simulink model "modelisation_nacelle_pour_tp_moteur_2015b"  (R2015b)
settings: Solver=VariableStepAuto  StartTime=0.0  StopTime=10  RelTol=1e-3
PreLoadFcn:
  | coef_ff=0.002
  | L=0.012
  | R=11
  | Ualim=7.2
  | kw=2e-2
  | p=7
  | echelon_roulis=10
  | echelon_tangage=10
  | kp_roulis=1000
  | ki_roulis=800
  | kd_roulis=0
  | kp_tangage=1000
  | ki_tangage=800
  | kd_tangage=0
  | pwm_max=127
undefined symbols (not defined in the file): sigbuilder_block, X, Y, Z
libraries: sm_lib x164, nesl_utility x5, simulink x1
(part 1 of 4)
settings Model: Creator=pt_ptsi  LastModifiedBy=Phil
settings SolverCC: ZeroCrossAlgorithm=Adaptive
settings DataIOCC: SaveFormat=Array
settings OptimizationCC: ExpressionDepthLimit=2147483647
settings DebuggingCC: UnderspecifiedInitializationDetection=Classic  MergeDetectMultiDrivingBlocksExec=none  SolverPrmCheckMsg=warning  StateNameClashWarn=warning
settings HardwareCC: ProdBitPerPointer=32  ProdLargestAtomicFloat=None  ProdIntDivRoundTo=Undefined  ProdEndianess=Unspecified  ProdWordSize=32  ProdHWDeviceType=32-bit Generic
settings GRTTargetCC: GeneratePreprocessorConditionals=Disable all
settings ConfigComp: CovModelRefEnable=Off
settings ExplorerConfigSet: SimMechanicsOpenEditorOnUpdate=off  InternalSimMechanicsExplorerSettings="<ExplorerConfiguration><canonicalview>default</canonicalview><AnimationSetting><BasePlaybackSpeed>1.0</BasePlaybackSpeed><PlaybackSpeedFactor>1.0</PlaybackSpeedFactor></AnimationSetting><TilePanel><TileInfo><Tiles Columns=\"1\" Count=\"1\" Rows=\"1\"><Column Left=\"2\" Weight=\"1\"/><Column Left=\"662\"/><Row Top=\"2\" Weight=\"1\"/><Row Top=\"396\"/><Tile Height=\"1\" Width=\"1\" X=\"0\" Y=\"0\"/></Tiles></TileInfo><SceneInfo><SceneViewer><BGColor><R>0.60000002384185791</R><G>0.60000002384185791</G><B>0.60000002384185791</B></BGColor><Camera><DoPerspective>off</DoPerspective><Position><X>12.213943667440395</X><Y>12.912141479051609</Y><Z>-9.9128663307728146</Z></Position><Center><X>0.0036568356529240731</X><Y>0.0029282546692730449</Y><Z>-0.080202307970983711</Z></Center><Up><X>0.79405149944444098</X><Y>-0.40757170789975361</Y><Z>0.45096288001310419</Z></Up><ViewLimDist>1</ViewLimDist><YLim>0.061319680660963063</YLim><XLim>0.10368600548126482</XLim></Camera></SceneViewer></SceneInfo></TilePanel><MechEditorPanel><Cameras/><GfxPanelCameraMap/></MechEditorPanel></ExplorerConfiguration>"

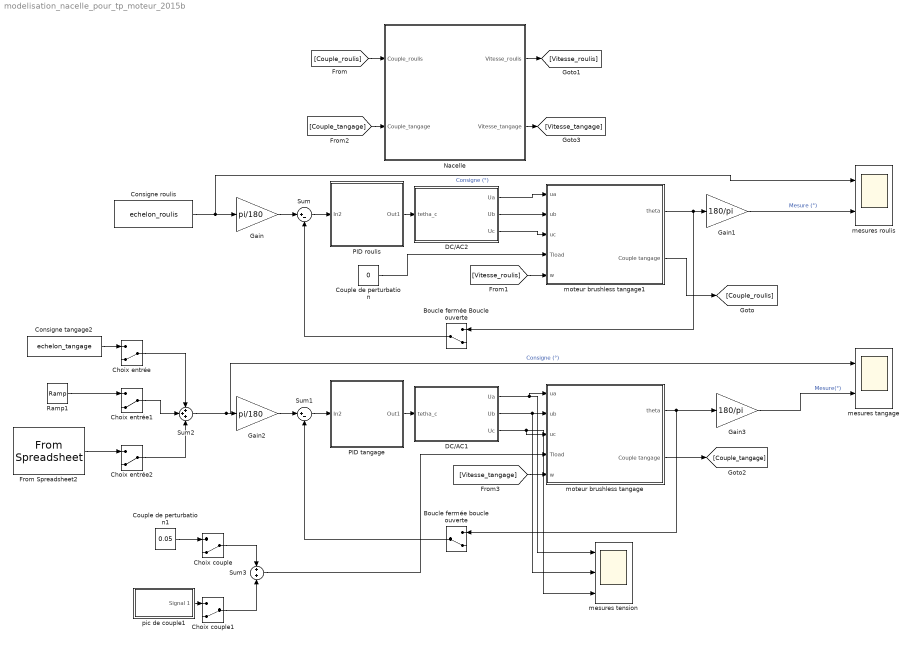
== system modelisation_nacelle_pour_tp_moteur_2015b ==
  Boucle fermée Boucle ouverte : ManualSwitch  CurrentSetting=0
  Boucle fermée boucle ouverte : ManualSwitch  CurrentSetting=0
  Choix couple : ManualSwitch  CurrentSetting=0
  Choix couple1 : ManualSwitch  CurrentSetting=0
  Choix entrée : ManualSwitch  CurrentSetting=0
  Choix entrée1 : ManualSwitch  CurrentSetting=0
  Choix entrée2 : ManualSwitch  CurrentSetting=0
  Consigne roulis : Constant  Value=echelon_roulis
  Consigne tangage2 : Constant  Value=echelon_tangage
  Couple de perturbation : Constant  Value=0
  Couple de perturbation1 : Constant  Value=0.05
  DC/AC1 : Subsystem
      mask Display: image('DC_AC.bmp')
  DC/AC2 : Subsystem
      mask Display: image('DC_AC.bmp')
  From Spreadsheet2 : FromSpreadsheet  FileName=pos.xlsx  SheetName=Feuil1
  Gain : Gain  Gain=pi/180
  Gain1 : Gain  Gain=180/pi
  Gain2 : Gain  Gain=pi/180
  Gain3 : Gain  Gain=180/pi
  Nacelle : Subsystem
      mask Display: image('image_nacelle.bmp')
  PID roulis : Subsystem
      mask Display: image('image PID.bmp')
  PID tangage : Subsystem
      mask Display: image('image PID.bmp')
  Ramp1 : simulink/Sources/Ramp  slope=100  start=0  X0=0
  Sum : Sum  Inputs=|+-
  Sum1 : Sum  Inputs=|+-
  Sum2 : Sum  Inputs=+++
  Sum3 : Sum
  mesures roulis : Scope  NumInputPorts=2
  mesures tangage : Scope  NumInputPorts=2
  mesures tension : Scope  NumInputPorts=3
  moteur brushless tangage : Subsystem
      mask Display: image('moteurBL.jpg')
  moteur brushless tangage1 : Subsystem
      mask Display: image('moteurBL.jpg')
  pic de couple1 : Subsystem  Tag=STV Subsys  LoadFcn=sigbuilder_block('load');  StartFcn=sigbuilder_block('start');  StopFcn=sigbuilder_block('stop');  ClipboardFcn=sigbuilder_block('clipboard');  mask(Sigbuilder block){}
      mask help: Simulink:masks:SigbuilderBlock_MD
      mask init:
      | if ~strcmp(get_param(bdroot(gcbh),'SimulationStatus'),'stopped') tuvar = sigbuilder_block('maskInit'); end
      settings: CopyFcn=sigbuilder_block('copy');  DeleteFcn=sigbuilder_block('delete');  ModelCloseFcn=sigbuilder_block('modelClose');  PreSaveFcn=sigbuilder_block('preSave');  PauseFcn=sigbuilder_block('pause');  ContinueFcn=sigbuilder_block('continue');  NameChangeFcn=sigbuilder_block('namechange');  OpenFcn=sigbuilder_block('open',[6 30 1428 682.5 ]);  CloseFcn=sigbuilder_block('close');
      mask Display: plot(0, 0, 100, 100,[2, 2, 32, 32, 2], [68, 8, 8, 68, 68],[32, 2], [38, 38], [32, 19, 2],[53, 60, 44], [32, 17, 17, 2],[16, 16, 31, 31]);txt = getActiveGroup(gcbh);text(2, 100, txt,'verticalAlignment', 'top');
  wires:
  DC/AC2/1(Ua) -> moteur brushless tangage1/1(ua)
  DC/AC2/2(Ub) -> moteur brushless tangage1/2(ub)
  DC/AC2/3(Uc) -> moteur brushless tangage1/3(uc)
  Couple de perturbation/1 -> moteur brushless tangage1/4(Tload)
  Gain/1 -> Sum/1
  moteur brushless tangage1/1(theta) -> Boucle fermée Boucle ouverte/1, Gain1/1
  Boucle fermée Boucle ouverte/1 -> Sum/2
  Consigne roulis/1 -> Gain/1, mesures roulis/1  "Consigne (°)"
  Gain1/1 -> mesures roulis/2  "Mesure (°)"
  Sum/1 -> PID roulis/1(In2)
  PID roulis/1(Out1) -> DC/AC2/1(tetha_c)
  Gain2/1 -> Sum1/1
  moteur brushless tangage/1(theta) -> Boucle fermée boucle ouverte/1, Gain3/1
  Boucle fermée boucle ouverte/1 -> Sum1/2
  Sum2/1 -> Gain2/1, mesures tangage/1  "Consigne (°)"
  Gain3/1 -> mesures tangage/2  "Mesure(°)"
  DC/AC1/1(Ua) -> mesures tension/1, moteur brushless tangage/1(ua)
  DC/AC1/2(Ub) -> mesures tension/2, moteur brushless tangage/2(ub)
  DC/AC1/3(Uc) -> mesures tension/3, moteur brushless tangage/3(uc)
  Sum1/1 -> PID tangage/1(In2)
  PID tangage/1(Out1) -> DC/AC1/1(tetha_c)
  moteur brushless tangage1/2(Couple tangage) -> [Couple_roulis]
  [Couple_roulis] -> Nacelle/1(Couple_roulis)
  [Vitesse_roulis] -> moteur brushless tangage1/5(w)
  Nacelle/1(Vitesse_roulis) -> [Vitesse_roulis]
  moteur brushless tangage/2(Couple tangage) -> [Couple_tangage]
  [Couple_tangage] -> Nacelle/2(Couple_tangage)
  Nacelle/2(Vitesse_tangage) -> [Vitesse_tangage]
  [Vitesse_tangage] -> moteur brushless tangage/5(w)
  Sum3/1 -> moteur brushless tangage/4(Tload)
  Consigne tangage2/1 -> Choix entrée/1
  Ramp1/1 -> Choix entrée1/1
  From Spreadsheet2/1 -> Choix entrée2/1
  Choix entrée/1 -> Sum2/1
  Choix entrée1/1 -> Sum2/2
  Choix entrée2/1 -> Sum2/3
  Couple de perturbation1/1 -> Choix couple/1
  pic de couple1/1(Signal 1) -> Choix couple1/1
  Choix couple1/1 -> Sum3/2
  Choix couple/1 -> Sum3/1

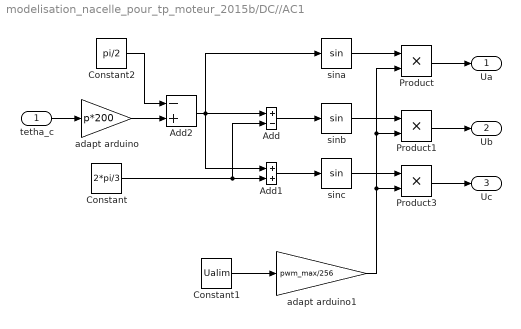
== system modelisation_nacelle_pour_tp_moteur_2015b/DC//AC1 ==
  tetha_c : Inport
  Add : Sum  Inputs=+-
  Add1 : Sum
  Add2 : Sum  Inputs=-+
  Constant : Constant  Value=2*pi/3
  Constant1 : Constant  Value=Ualim
  Constant2 : Constant  Value=pi/2
  Product : Product  RndMeth=Zero
  Product1 : Product  RndMeth=Zero
  Product3 : Product  RndMeth=Zero
  adapt arduino : Gain  Gain=p*200
  adapt arduino1 : Gain  Gain=pwm_max/256
  sina : Trigonometry
  sinb : Trigonometry
  sinc : Trigonometry
  Ua : Outport
  Ub : Outport  Port=2
  Uc : Outport  Port=3
  wires:
  tetha_c/1 -> adapt arduino/1
  Add2/1 -> sina/1, Add/1, Add1/1
  Constant2/1 -> Add2/1
  sinc/1 -> Product3/1
  sinb/1 -> Product1/1
  Product3/1 -> Uc/1
  Product1/1 -> Ub/1
  Product/1 -> Ua/1
  sina/1 -> Product/1
  Constant/1 -> Add1/2, Add/2
  Add/1 -> sinb/1
  Add1/1 -> sinc/1
  adapt arduino/1 -> Add2/2
  Constant1/1 -> adapt arduino1/1
  adapt arduino1/1 -> Product3/2, Product1/2, Product/2

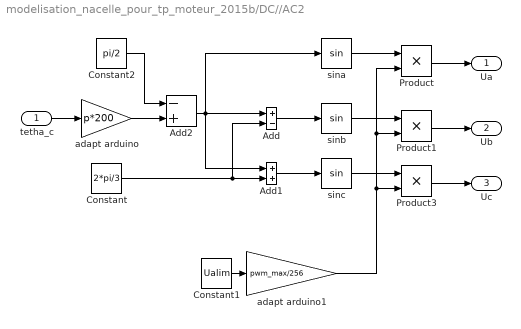
== system modelisation_nacelle_pour_tp_moteur_2015b/DC//AC2 ==
  tetha_c : Inport
  Add : Sum  Inputs=+-
  Add1 : Sum
  Add2 : Sum  Inputs=-+
  Constant : Constant  Value=2*pi/3
  Constant1 : Constant  Value=Ualim
  Constant2 : Constant  Value=pi/2
  Product : Product  RndMeth=Zero
  Product1 : Product  RndMeth=Zero
  Product3 : Product  RndMeth=Zero
  adapt arduino : Gain  Gain=p*200
  adapt arduino1 : Gain  Gain=pwm_max/256
  sina : Trigonometry
  sinb : Trigonometry
  sinc : Trigonometry
  Ua : Outport
  Ub : Outport  Port=2
  Uc : Outport  Port=3
  wires:
  adapt arduino1/1 -> Product/2, Product1/2, Product3/2
  Constant1/1 -> adapt arduino1/1
  adapt arduino/1 -> Add2/2
  Add1/1 -> sinc/1
  Add/1 -> sinb/1
  Constant/1 -> Add/2, Add1/2
  sina/1 -> Product/1
  Product/1 -> Ua/1
  Product1/1 -> Ub/1
  Product3/1 -> Uc/1
  sinb/1 -> Product1/1
  sinc/1 -> Product3/1
  Constant2/1 -> Add2/1
  Add2/1 -> Add1/1, Add/1, sina/1
  tetha_c/1 -> adapt arduino/1

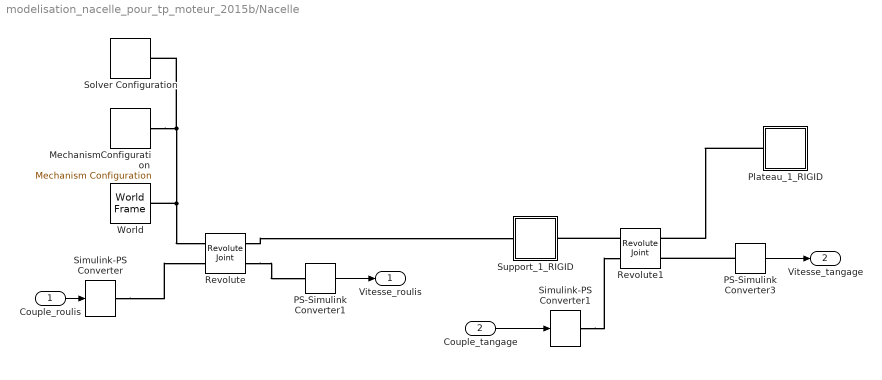
== system modelisation_nacelle_pour_tp_moteur_2015b/Nacelle ==
  Couple_roulis : Inport
  Couple_tangage : Inport  Port=2
  MechanismConfiguration : sm_lib/Utilities/Mechanism Configuration  UniformGravity=Constant  GravityVector=[0 0 0]  GravityUnits=m/s^2  LinearizationDelta=0.001
  PS-Simulink Converter1 : nesl_utility/PS-Simulink Converter  PhysicalDomain=network_engine_domain  SubClassName=ps_output  LeftPortType=input  RightPortType=output  PseudoPeriodic=off  Frequencies=[]  Unit=1  AffineConversion=off
  PS-Simulink Converter3 : nesl_utility/PS-Simulink Converter  PhysicalDomain=network_engine_domain  SubClassName=ps_output  LeftPortType=input  RightPortType=output  PseudoPeriodic=off  Frequencies=[]  Unit=1  AffineConversion=off
  Plateau_1_RIGID : Subsystem
  Revolute : sm_lib/Joints/Revolute Joint  SenseConstraintForce=off  SenseConstraintForceX=off  SenseConstraintForceY=off  SenseConstraintForceZ=off  SenseConstraintTorque=off  SenseConstraintTorqueX=off  SenseConstraintTorqueY=off  SenseConstraintTorqueZ=off  SenseTotalForce=off  SenseTotalForceX=off  SenseTotalForceY=off  SenseTotalForceZ=off  SenseTotalTorque=off  SenseTotalTorqueX=off  SenseTotalTorqueY=off  SenseTotalTorqueZ=off  CompositeWrenchDir=FollowerOnBase  CompositeWrenchFrame=BaseFrame  EquilibriumPosition=0  EquilibriumPositionUnits=rad  SpringStiffness=0  SpringStiffnessUnits=m*N/rad  DampingCoefficient=coef_ff  DampingCoefficientUnits=m*s*N/rad  TorqueActuationMode=InputTorque  MotionActuationMode=ComputedMotion  SensePosition=off  SenseVelocity=on  SenseAcceleration=off  SenseTorqueForce=off  PositionTargetSpecify=on  PositionTargetPriority=Low  PositionTargetValue=90  PositionTargetValueUnits=deg  VelocityTargetSpecify=off  VelocityTargetPriority=High  VelocityTargetValue=0  VelocityTargetValueUnits=deg/s
  Revolute1 : sm_lib/Joints/Revolute Joint  SenseConstraintForce=off  SenseConstraintForceX=off  SenseConstraintForceY=off  SenseConstraintForceZ=off  SenseConstraintTorque=off  SenseConstraintTorqueX=off  SenseConstraintTorqueY=off  SenseConstraintTorqueZ=off  SenseTotalForce=off  SenseTotalForceX=off  SenseTotalForceY=off  SenseTotalForceZ=off  SenseTotalTorque=off  SenseTotalTorqueX=off  SenseTotalTorqueY=off  SenseTotalTorqueZ=off  CompositeWrenchDir=FollowerOnBase  CompositeWrenchFrame=BaseFrame  EquilibriumPosition=0  EquilibriumPositionUnits=rad  SpringStiffness=0  SpringStiffnessUnits=m*N/rad  DampingCoefficient=coef_ff  DampingCoefficientUnits=m*s*N/rad  TorqueActuationMode=InputTorque  MotionActuationMode=ComputedMotion  SensePosition=off  SenseVelocity=on  SenseAcceleration=off  SenseTorqueForce=off  PositionTargetSpecify=on  PositionTargetPriority=Low  PositionTargetValue=0180  PositionTargetValueUnits=deg  VelocityTargetSpecify=off  VelocityTargetPriority=High  VelocityTargetValue=0  VelocityTargetValueUnits=deg/s
  Simulink-PS Converter : nesl_utility/Simulink-PS Converter  PhysicalDomain=network_engine_domain  SubClassName=ps_input  LeftPortType=input  RightPortType=output  PseudoPeriodic=off  Frequencies=[]  NoiseDistribution=none  NoiseParameters=[]  Unit=1  AffineConversion=off  InputFiltering=off  SimscapeFilterOrder=1  InputFilterTimeConstant=0.001  UdotUserProvided=1
  Simulink-PS Converter1 : nesl_utility/Simulink-PS Converter  PhysicalDomain=network_engine_domain  SubClassName=ps_input  LeftPortType=input  RightPortType=output  PseudoPeriodic=off  Frequencies=[]  NoiseDistribution=none  NoiseParameters=[]  Unit=1  AffineConversion=off  InputFiltering=off  SimscapeFilterOrder=1  InputFilterTimeConstant=0.001  UdotUserProvided=1
  Solver Configuration : nesl_utility/Solver Configuration  PhysicalDomain=network_engine_domain  SubClassName=solver  LeftPortType=input  RightPortType=generic  Accelerate=off  Tones=[]  Harmonics=[]  SimulateNoise=off  Profile=off  UseLocalSampling=off  EnableSwitchedLinearOptims=on  FrequencyDomain=off  UseCCode=off  RelTol=0.001  AbsTol=1e-06  MinStep=1e-09  ToWorkspace=off  RevertToSquareIcSolve=off  NumHomotopyIterations=100  PhasorMode=off  PhasorModeNumHarmonics=1  OverrideAbsTol=off  DoDC=off  ResidualTolerance=1e-09  UseLocalSolver=off  LocalSolverChoice=NE_BACKWARD_EULER_ADVANCER  LocalSolverSampleTime=0.001  DoFixedCost=off  MaxNonlinIter=3  MaxModeIter=2  LinearAlgebra=Sparse  DelaysMemoryBudget=1024  AutomaticFiltering=on  FilteringTimeConstant=0.001
  Support_1_RIGID : Subsystem
  World : sm_lib/Frames and Transforms/World Frame
  Vitesse_roulis : Outport
  Vitesse_tangage : Outport  Port=2
  wires:
  Couple_roulis/1 -> Simulink-PS Converter/1
  PS-Simulink Converter1/1 -> Vitesse_roulis/1
  Couple_tangage/1 -> Simulink-PS Converter1/1
  PS-Simulink Converter3/1 -> Vitesse_tangage/1
  connections:
  Revolute/RConn1 -- Support_1_RIGID/LConn1
  Revolute1/LConn1 -- Support_1_RIGID/RConn1
  Plateau_1_RIGID/LConn1 -- Revolute1/RConn1
  MechanismConfiguration/RConn1 -- Solver Configuration/RConn1 -- Revolute/LConn1 -- World/RConn1
  Simulink-PS Converter/RConn1 -- Revolute/LConn2
  Revolute/RConn2 -- PS-Simulink Converter1/LConn1
  PS-Simulink Converter3/LConn1 -- Revolute1/RConn2
  Simulink-PS Converter1/RConn1 -- Revolute1/LConn2

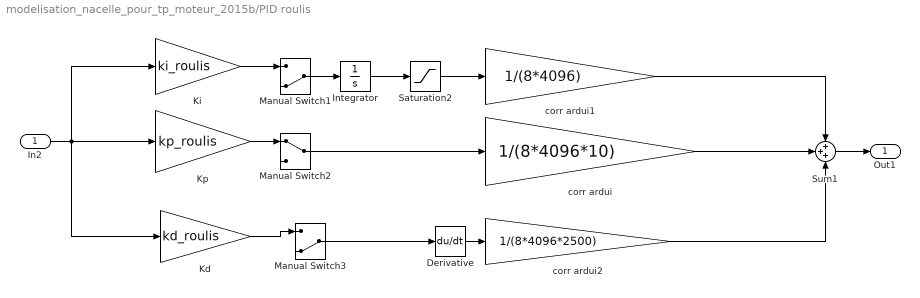
== system modelisation_nacelle_pour_tp_moteur_2015b/PID roulis ==
  In2 : Inport
  Derivative : Derivative
  Integrator : Integrator
  Kd : Gain  Gain=kd_roulis
  Ki : Gain  Gain=ki_roulis
  Kp : Gain  Gain=kp_roulis
  Manual Switch1 : ManualSwitch  CurrentSetting=0
  Manual Switch2 : ManualSwitch
  Manual Switch3 : ManualSwitch  CurrentSetting=0
  Saturation2 : Saturate  UpperLimit=100000  LowerLimit=-100000
  Sum1 : Sum  Inputs=+++
  corr ardui : Gain  Gain=1/(8*4096*10)
  corr ardui1 : Gain  Gain=1/(8*4096)
  corr ardui2 : Gain  Gain=1/(8*4096*2500)
  Out1 : Outport
  wires:
  In2/1 -> Ki/1, Kd/1, Kp/1
  corr ardui1/1 -> Sum1/1
  Sum1/1 -> Out1/1
  Kp/1 -> Manual Switch2/1
  Manual Switch1/1 -> Integrator/1
  Ki/1 -> Manual Switch1/1
  Derivative/1 -> corr ardui2/1
  corr ardui2/1 -> Sum1/3
  Integrator/1 -> Saturation2/1
  corr ardui/1 -> Sum1/2
  Manual Switch3/1 -> Derivative/1
  Manual Switch2/1 -> corr ardui/1
  Kd/1 -> Manual Switch3/1
  Saturation2/1 -> corr ardui1/1

== system modelisation_nacelle_pour_tp_moteur_2015b/PID tangage ==
  In2 : Inport
  Derivative : Derivative
  Integrator : Integrator
  Kd : Gain  Gain=kd_tangage
  Ki : Gain  Gain=ki_tangage
  Kp : Gain  Gain=kp_tangage
  Manual Switch1 : ManualSwitch  CurrentSetting=0
  Manual Switch2 : ManualSwitch
  Manual Switch3 : ManualSwitch  CurrentSetting=0
  Saturation2 : Saturate  UpperLimit=100000  LowerLimit=-100000
  Sum1 : Sum  Inputs=+++
  corr ardui : Gain  Gain=1/(8*4096*10)
  corr ardui1 : Gain  Gain=1/(8*4096)
  corr ardui2 : Gain  Gain=1/(8*4096*2500)
  Out1 : Outport
  wires:
  Kd/1 -> Manual Switch3/1
  Manual Switch2/1 -> corr ardui/1
  Manual Switch3/1 -> Derivative/1
  corr ardui/1 -> Sum1/2
  Integrator/1 -> Saturation2/1
  corr ardui2/1 -> Sum1/3
  Derivative/1 -> corr ardui2/1
  Ki/1 -> Manual Switch1/1
  Manual Switch1/1 -> Integrator/1
  Kp/1 -> Manual Switch2/1
  Sum1/1 -> Out1/1
  corr ardui1/1 -> Sum1/1
  In2/1 -> Kd/1, Kp/1, Ki/1
  Saturation2/1 -> corr ardui1/1

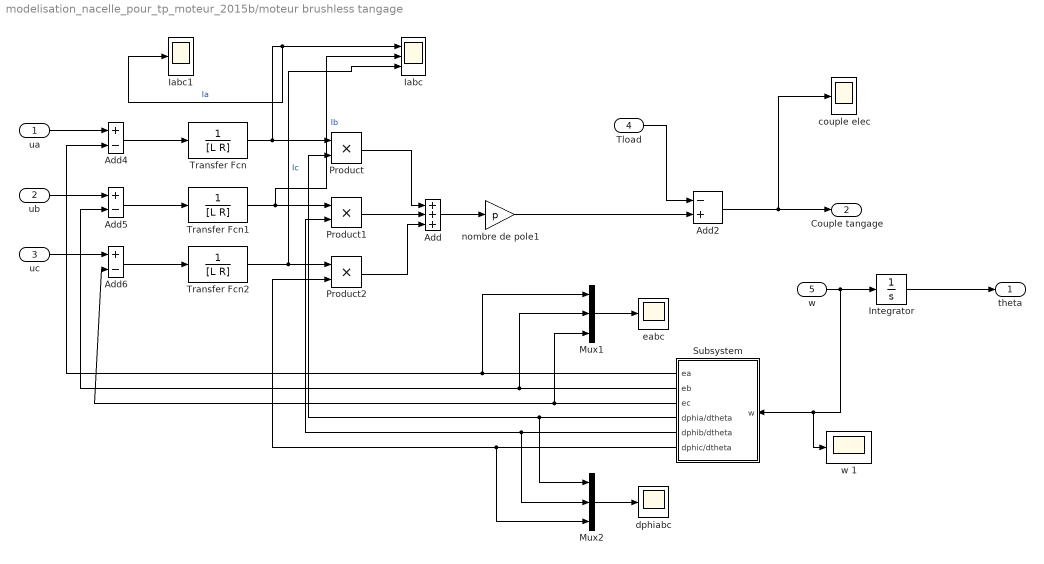
== system modelisation_nacelle_pour_tp_moteur_2015b/moteur brushless tangage ==
  ua : Inport
  ub : Inport  Port=2
  uc : Inport  Port=3
  Tload : Inport  Port=4
  w : Inport  Port=5
  Add : Sum  Inputs=+++
  Add2 : Sum  Inputs=-+
  Add4 : Sum  Inputs=+-
  Add5 : Sum  Inputs=+-
  Add6 : Sum  Inputs=+-
  Iabc : Scope  NumInputPorts=3
  Iabc1 : Scope
  Integrator : Integrator
  Mux1 : Mux  Inputs=3
  Mux2 : Mux  Inputs=3
  Product : Product  RndMeth=Zero
  Product1 : Product  RndMeth=Zero
  Product2 : Product  RndMeth=Zero
  Subsystem : Subsystem
  Transfer Fcn : TransferFcn  Denominator=[L R]
  Transfer Fcn1 : TransferFcn  Denominator=[L R]
  Transfer Fcn2 : TransferFcn  Denominator=[L R]
  couple elec : Scope
  dphiabc : Scope
  "eabc " : Scope
  nombre de pole1 : Gain  Gain=p
  w 1 : Scope
  theta : Outport
  Couple tangage : Outport  Port=2
  wires:
  nombre de pole1/1 -> Add2/2
  Add2/1 -> Couple tangage/1, couple elec/1
  ua/1 -> Add4/1
  w/1 -> Integrator/1, Subsystem/1(w), w 1/1
  Mux2/1 -> dphiabc/1
  Integrator/1 -> theta/1
  Subsystem/6(dphic/dtheta) -> Product2/2, Mux2/3
  Subsystem/5(dphib/dtheta) -> Product1/2, Mux2/2
  Subsystem/4(dphia/dtheta) -> Product/2, Mux2/1
  Mux1/1 -> "eabc "/1
  Transfer Fcn2/1 -> Iabc/3, Product2/1  "Ic"
  Add6/1 -> Transfer Fcn2/1
  Add5/1 -> Transfer Fcn1/1
  Product1/1 -> Add/2
  Product2/1 -> Add/3
  Add4/1 -> Transfer Fcn/1
  Add/1 -> nombre de pole1/1
  Transfer Fcn/1 -> Iabc1/1, Iabc/1, Product/1  "Ia"
  Transfer Fcn1/1 -> Iabc/2, Product1/1  "Ib"
  Product/1 -> Add/1
  uc/1 -> Add6/1
  ub/1 -> Add5/1
  Tload/1 -> Add2/1
  Subsystem/3(ec) -> Add6/2, Mux1/3
  Subsystem/1(ea) -> Add4/2, Mux1/1
  Subsystem/2(eb) -> Add5/2, Mux1/2

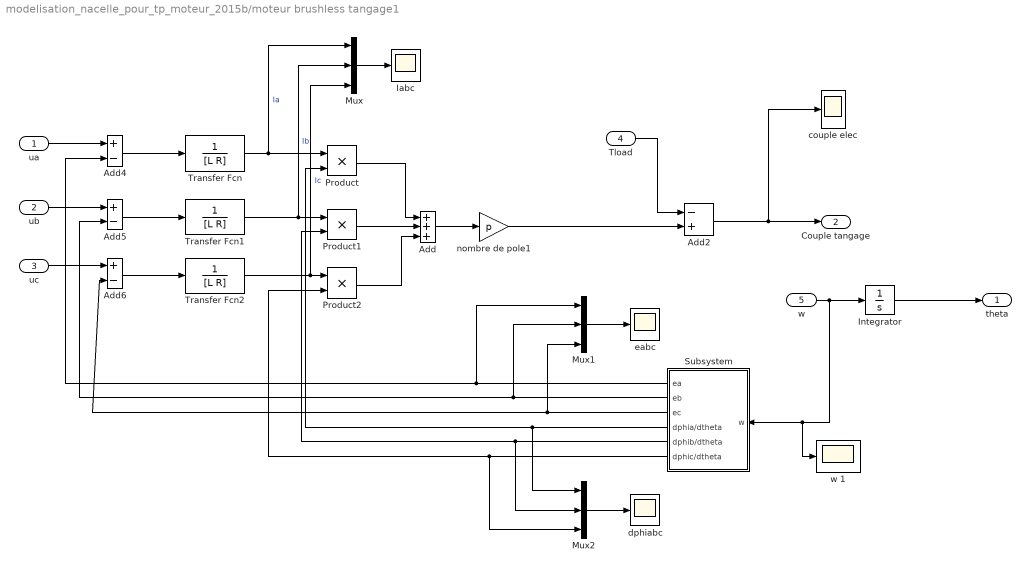
== system modelisation_nacelle_pour_tp_moteur_2015b/moteur brushless tangage1 ==
  ua : Inport
  ub : Inport  Port=2
  uc : Inport  Port=3
  Tload : Inport  Port=4
  w : Inport  Port=5
  Add : Sum  Inputs=+++
  Add2 : Sum  Inputs=-+
  Add4 : Sum  Inputs=+-
  Add5 : Sum  Inputs=+-
  Add6 : Sum  Inputs=+-
  Iabc : Scope
  Integrator : Integrator
  Mux : Mux  Inputs=3
  Mux1 : Mux  Inputs=3
  Mux2 : Mux  Inputs=3
  Product : Product  RndMeth=Zero
  Product1 : Product  RndMeth=Zero
  Product2 : Product  RndMeth=Zero
  Subsystem : Subsystem
  Transfer Fcn : TransferFcn  Denominator=[L R]
  Transfer Fcn1 : TransferFcn  Denominator=[L R]
  Transfer Fcn2 : TransferFcn  Denominator=[L R]
  couple elec : Scope
  dphiabc : Scope
  "eabc " : Scope
  nombre de pole1 : Gain  Gain=p
  w 1 : Scope
  theta : Outport
  Couple tangage : Outport  Port=2
  wires:
  nombre de pole1/1 -> Add2/2
  Add2/1 -> Couple tangage/1, couple elec/1
  ua/1 -> Add4/1
  w/1 -> Integrator/1, Subsystem/1(w), w 1/1
  Mux2/1 -> dphiabc/1
  Integrator/1 -> theta/1
  Subsystem/6(dphic/dtheta) -> Product2/2, Mux2/3
  Subsystem/5(dphib/dtheta) -> Product1/2, Mux2/2
  Subsystem/4(dphia/dtheta) -> Product/2, Mux2/1
  Mux1/1 -> "eabc "/1
  Mux/1 -> Iabc/1
  Transfer Fcn2/1 -> Product2/1, Mux/3  "Ic"
  Add6/1 -> Transfer Fcn2/1
  Add5/1 -> Transfer Fcn1/1
  Product1/1 -> Add/2
  Product2/1 -> Add/3
  Add4/1 -> Transfer Fcn/1
  Add/1 -> nombre de pole1/1
  Transfer Fcn/1 -> Product/1, Mux/1  "Ia"
  Transfer Fcn1/1 -> Product1/1, Mux/2  "Ib"
  Product/1 -> Add/1
  uc/1 -> Add6/1
  ub/1 -> Add5/1
  Tload/1 -> Add2/1
  Subsystem/3(ec) -> Add6/2, Mux1/3
  Subsystem/1(ea) -> Add4/2, Mux1/1
  Subsystem/2(eb) -> Add5/2, Mux1/2

== system modelisation_nacelle_pour_tp_moteur_2015b/pic de couple1 ==
  Demux : Demux  Tag=STV Demux  Outputs=1
  FromWs : FromWorkspace  Tag=STV FromWs  VariableName=tuvar  SampleTime=0
      SigBuilderData=|
      | common.afterFinalStr = 'Extrapolate'
      | common.sampleTime = 0
      | dataSet.timeRange = [0 10]
      | dataSet.name = 'Group 1'
      | sbobj.Groups.Name = 'Group 1'
      | sbobj.Groups.Signals.Name = 'Signal 1'
      | sbobj.Groups.Signals.XData = [0 1 1 1.02 1.03 2 2 2.05 2.05 10]
      | sbobj.Groups.Signals.YData = [0 0 0.1 0.1 0 0 -0.1 -0.1 0 0]
  Signal 1 : Outport  Tag=STV Outport
  wires:
  Demux/1 -> Signal 1/1
  FromWs/1 -> Demux/1

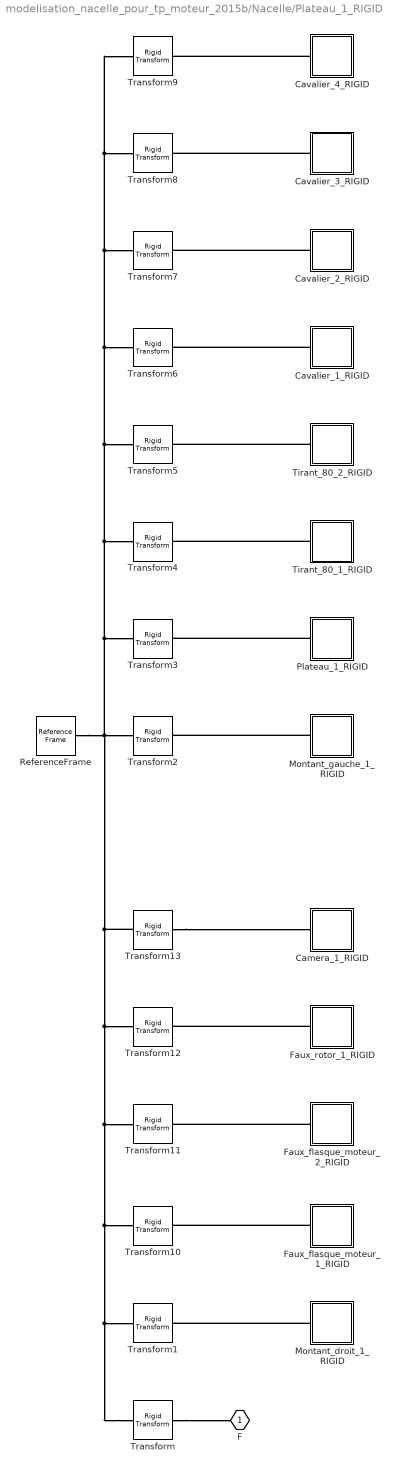
== system modelisation_nacelle_pour_tp_moteur_2015b/Nacelle/Plateau_1_RIGID ==
  Camera_1_RIGID : Subsystem
  Cavalier_1_RIGID : Subsystem
  Cavalier_2_RIGID : Subsystem
  Cavalier_3_RIGID : Subsystem
  Cavalier_4_RIGID : Subsystem
  Faux_flasque_moteur_1_RIGID : Subsystem
  Faux_flasque_moteur_2_RIGID : Subsystem
  Faux_rotor_1_RIGID : Subsystem
  Montant_droit_1_RIGID : Subsystem
  Montant_gauche_1_RIGID : Subsystem
  Plateau_1_RIGID : Subsystem
  ReferenceFrame : sm_lib/Frames and Transforms/Reference Frame
  Tirant_80_1_RIGID : Subsystem
  Tirant_80_2_RIGID : Subsystem
  Transform : sm_lib/Frames and Transforms/Rigid Transform  TranslationMethod=Cartesian  TranslationLengthUnit=mm  TranslationStandardAxis=+Z  TranslationStandardOffset=0  TranslationCartesianOffset=[-86.186770000000294 -350.63886829239681 59.075438580129507]  TranslationROffset=0  TranslationROffsetUnits=m  TranslationZOffset=0  TranslationZOffsetUnits=m  TranslationThetaOffset=0  TranslationThetaOffsetUnits=deg  RotationMethod=ArbitraryAxis  RotationAngleUnits=rad  RotationStandardAxis=+Z  RotationAngle=2.0943951023931926  RotationArbitraryAxis=[-0.57735026918962473 -0.57735026918962473 0.57735026918962795]  FollAlignAxisA=+X  BaseAlignAxisA=+Y  FollAlignAxisB=+Y  BaseAlignAxisB=+Z  RotationSequenceAxes=FollowerAxes  RotationSequence=XYX  RotationSequenceAngles=[0 0 0]  RotationSequenceAnglesUnits=deg  RotationMatrix=[1 0 0; 0 1 0; 0 0 1]
  Transform1 : sm_lib/Frames and Transforms/Rigid Transform  TranslationMethod=Cartesian  TranslationLengthUnit=mm  TranslationStandardAxis=+Z  TranslationStandardOffset=0  TranslationCartesianOffset=[43 -350.63899999999995 59.075700000000005]  TranslationROffset=0  TranslationROffsetUnits=m  TranslationZOffset=0  TranslationZOffsetUnits=m  TranslationThetaOffset=0  TranslationThetaOffsetUnits=deg  RotationMethod=ArbitraryAxis  RotationAngleUnits=rad  RotationStandardAxis=+Z  RotationAngle=1.5707963267948968  RotationArbitraryAxis=[0 1 0]  FollAlignAxisA=+X  BaseAlignAxisA=+Y  FollAlignAxisB=+Y  BaseAlignAxisB=+Z  RotationSequenceAxes=FollowerAxes  RotationSequence=XYX  RotationSequenceAngles=[0 0 0]  RotationSequenceAnglesUnits=deg  RotationMatrix=[1 0 0; 0 1 0; 0 0 1]
  Transform10 : sm_lib/Frames and Transforms/Rigid Transform  TranslationMethod=Cartesian  TranslationLengthUnit=mm  TranslationStandardAxis=+Z  TranslationStandardOffset=0  TranslationCartesianOffset=[-43 -350.63899999999995 59.075700000000005]  TranslationROffset=0  TranslationROffsetUnits=m  TranslationZOffset=0  TranslationZOffsetUnits=m  TranslationThetaOffset=0  TranslationThetaOffsetUnits=deg  RotationMethod=ArbitraryAxis  RotationAngleUnits=rad  RotationStandardAxis=+Z  RotationAngle=0.1267884277623974  RotationArbitraryAxis=[1 -5.2973056331010912e-15 0]  FollAlignAxisA=+X  BaseAlignAxisA=+Y  FollAlignAxisB=+Y  BaseAlignAxisB=+Z  RotationSequenceAxes=FollowerAxes  RotationSequence=XYX  RotationSequenceAngles=[0 0 0]  RotationSequenceAnglesUnits=deg  RotationMatrix=[1 0 0; 0 1 0; 0 0 1]
  Transform11 : sm_lib/Frames and Transforms/Rigid Transform  TranslationMethod=Cartesian  TranslationLengthUnit=mm  TranslationStandardAxis=+Z  TranslationStandardOffset=0  TranslationCartesianOffset=[43 -350.63899999999995 59.075700000000005]  TranslationROffset=0  TranslationROffsetUnits=m  TranslationZOffset=0  TranslationZOffsetUnits=m  TranslationThetaOffset=0  TranslationThetaOffsetUnits=deg  RotationMethod=ArbitraryAxis  RotationAngleUnits=rad  RotationStandardAxis=+Z  RotationAngle=3.1415926535897931  RotationArbitraryAxis=[0 -0.063351760689794798 0.99799125968993485]  FollAlignAxisA=+X  BaseAlignAxisA=+Y  FollAlignAxisB=+Y  BaseAlignAxisB=+Z  RotationSequenceAxes=FollowerAxes  RotationSequence=XYX  RotationSequenceAngles=[0 0 0]  RotationSequenceAnglesUnits=deg  RotationMatrix=[1 0 0; 0 1 0; 0 0 1]
  Transform12 : sm_lib/Frames and Transforms/Rigid Transform  TranslationMethod=Cartesian  TranslationLengthUnit=mm  TranslationStandardAxis=+Z  TranslationStandardOffset=0  TranslationCartesianOffset=[-47 -350.63899999999995 59.075700000000005]  TranslationROffset=0  TranslationROffsetUnits=m  TranslationZOffset=0  TranslationZOffsetUnits=m  TranslationThetaOffset=0  TranslationThetaOffsetUnits=deg  RotationMethod=ArbitraryAxis  RotationAngleUnits=rad  RotationStandardAxis=+Z  RotationAngle=0.1267884277623974  RotationArbitraryAxis=[1 -5.9793592673726155e-15 0]  FollAlignAxisA=+X  BaseAlignAxisA=+Y  FollAlignAxisB=+Y  BaseAlignAxisB=+Z  RotationSequenceAxes=FollowerAxes  RotationSequence=XYX  RotationSequenceAngles=[0 0 0]  RotationSequenceAnglesUnits=deg  RotationMatrix=[1 0 0; 0 1 0; 0 0 1]
  Transform13 : sm_lib/Frames and Transforms/Rigid Transform  TranslationMethod=Cartesian  TranslationLengthUnit=mm  TranslationStandardAxis=+Z  TranslationStandardOffset=0  TranslationCartesianOffset=[0 -340.63900000000001 71.075700000000012]  TranslationROffset=0  TranslationROffsetUnits=m  TranslationZOffset=0  TranslationZOffsetUnits=m  TranslationThetaOffset=0  TranslationThetaOffsetUnits=deg  RotationMethod=ArbitraryAxis  RotationAngleUnits=rad  RotationStandardAxis=+Z  RotationAngle=3.1415926535897922  RotationArbitraryAxis=[0 1 0]  FollAlignAxisA=+X  BaseAlignAxisA=+Y  FollAlignAxisB=+Y  BaseAlignAxisB=+Z  RotationSequenceAxes=FollowerAxes  RotationSequence=XYX  RotationSequenceAngles=[0 0 0]  RotationSequenceAnglesUnits=deg  RotationMatrix=[1 0 0; 0 1 0; 0 0 1]
  Transform2 : sm_lib/Frames and Transforms/Rigid Transform  TranslationMethod=Cartesian  TranslationLengthUnit=mm  TranslationStandardAxis=+Z  TranslationStandardOffset=0  TranslationCartesianOffset=[-40 -350.63899999999995 59.075700000000005]  TranslationROffset=0  TranslationROffsetUnits=m  TranslationZOffset=0  TranslationZOffsetUnits=m  TranslationThetaOffset=0  TranslationThetaOffsetUnits=deg  RotationMethod=ArbitraryAxis  RotationAngleUnits=rad  RotationStandardAxis=+Z  RotationAngle=1.570796326794897  RotationArbitraryAxis=[-0 -1 -0]  FollAlignAxisA=+X  BaseAlignAxisA=+Y  FollAlignAxisB=+Y  BaseAlignAxisB=+Z  RotationSequenceAxes=FollowerAxes  RotationSequence=XYX  RotationSequenceAngles=[0 0 0]  RotationSequenceAnglesUnits=deg  RotationMatrix=[1 0 0; 0 1 0; 0 0 1]
  Transform3 : sm_lib/Frames and Transforms/Rigid Transform  TranslationMethod=Cartesian  TranslationLengthUnit=mm  TranslationStandardAxis=+Z  TranslationStandardOffset=0  TranslationCartesianOffset=[0 -379.13900000000001 59.075700000000005]  TranslationROffset=0  TranslationROffsetUnits=m  TranslationZOffset=0  TranslationZOffsetUnits=m  TranslationThetaOffset=0  TranslationThetaOffsetUnits=deg  RotationMethod=ArbitraryAxis  RotationAngleUnits=rad  RotationStandardAxis=+Z  RotationAngle=2.0943951023931953  RotationArbitraryAxis=[-0.57735026918962584 0.57735026918962584 0.57735026918962584]  FollAlignAxisA=+X  BaseAlignAxisA=+Y  FollAlignAxisB=+Y  BaseAlignAxisB=+Z  RotationSequenceAxes=FollowerAxes  RotationSequence=XYX  RotationSequenceAngles=[0 0 0]  RotationSequenceAnglesUnits=deg  RotationMatrix=[1 0 0; 0 1 0; 0 0 1]
  Transform4 : sm_lib/Frames and Transforms/Rigid Transform  TranslationMethod=Cartesian  TranslationLengthUnit=mm  TranslationStandardAxis=+Z  TranslationStandardOffset=0  TranslationCartesianOffset=[-40 -373.13900000000001 73.075699999999998]  TranslationROffset=0  TranslationROffsetUnits=m  TranslationZOffset=0  TranslationZOffsetUnits=m  TranslationThetaOffset=0  TranslationThetaOffsetUnits=deg  RotationMethod=None  RotationAngleUnits=deg  RotationStandardAxis=+Z  RotationAngle=0  RotationArbitraryAxis=[0 0 1]  FollAlignAxisA=+X  BaseAlignAxisA=+Y  FollAlignAxisB=+Y  BaseAlignAxisB=+Z  RotationSequenceAxes=FollowerAxes  RotationSequence=XYX  RotationSequenceAngles=[0 0 0]  RotationSequenceAnglesUnits=deg  RotationMatrix=[1 0 0; 0 1 0; 0 0 1]
  Transform5 : sm_lib/Frames and Transforms/Rigid Transform  TranslationMethod=Cartesian  TranslationLengthUnit=mm  TranslationStandardAxis=+Z  TranslationStandardOffset=0  TranslationCartesianOffset=[-40 -373.13900000000001 45.075700000000005]  TranslationROffset=0  TranslationROffsetUnits=m  TranslationZOffset=0  TranslationZOffsetUnits=m  TranslationThetaOffset=0  TranslationThetaOffsetUnits=deg  RotationMethod=ArbitraryAxis  RotationAngleUnits=rad  RotationStandardAxis=+Z  RotationAngle=1.1076805483509773  RotationArbitraryAxis=[-1 0 0]  FollAlignAxisA=+X  BaseAlignAxisA=+Y  FollAlignAxisB=+Y  BaseAlignAxisB=+Z  RotationSequenceAxes=FollowerAxes  RotationSequence=XYX  RotationSequenceAngles=[0 0 0]  RotationSequenceAnglesUnits=deg  RotationMatrix=[1 0 0; 0 1 0; 0 0 1]
  Transform6 : sm_lib/Frames and Transforms/Rigid Transform  TranslationMethod=Cartesian  TranslationLengthUnit=mm  TranslationStandardAxis=+Z  TranslationStandardOffset=0  TranslationCartesianOffset=[25.5 -379.13900000000001 45.075700000000005]  TranslationROffset=0  TranslationROffsetUnits=m  TranslationZOffset=0  TranslationZOffsetUnits=m  TranslationThetaOffset=0  TranslationThetaOffsetUnits=deg  RotationMethod=ArbitraryAxis  RotationAngleUnits=rad  RotationStandardAxis=+Z  RotationAngle=1.5707963267948968  RotationArbitraryAxis=[0 1 0]  FollAlignAxisA=+X  BaseAlignAxisA=+Y  FollAlignAxisB=+Y  BaseAlignAxisB=+Z  RotationSequenceAxes=FollowerAxes  RotationSequence=XYX  RotationSequenceAngles=[0 0 0]  RotationSequenceAnglesUnits=deg  RotationMatrix=[1 0 0; 0 1 0; 0 0 1]
  Transform7 : sm_lib/Frames and Transforms/Rigid Transform  TranslationMethod=Cartesian  TranslationLengthUnit=mm  TranslationStandardAxis=+Z  TranslationStandardOffset=0  TranslationCartesianOffset=[25.5 -379.13900000000001 73.075699999999998]  TranslationROffset=0  TranslationROffsetUnits=m  TranslationZOffset=0  TranslationZOffsetUnits=m  TranslationThetaOffset=0  TranslationThetaOffsetUnits=deg  RotationMethod=ArbitraryAxis  RotationAngleUnits=rad  RotationStandardAxis=+Z  RotationAngle=1.5707963267948968  RotationArbitraryAxis=[0 1 0]  FollAlignAxisA=+X  BaseAlignAxisA=+Y  FollAlignAxisB=+Y  BaseAlignAxisB=+Z  RotationSequenceAxes=FollowerAxes  RotationSequence=XYX  RotationSequenceAngles=[0 0 0]  RotationSequenceAnglesUnits=deg  RotationMatrix=[1 0 0; 0 1 0; 0 0 1]
  Transform8 : sm_lib/Frames and Transforms/Rigid Transform  TranslationMethod=Cartesian  TranslationLengthUnit=mm  TranslationStandardAxis=+Z  TranslationStandardOffset=0  TranslationCartesianOffset=[-25.5 -379.13900000000001 45.075700000000005]  TranslationROffset=0  TranslationROffsetUnits=m  TranslationZOffset=0  TranslationZOffsetUnits=m  TranslationThetaOffset=0  TranslationThetaOffsetUnits=deg  RotationMethod=ArbitraryAxis  RotationAngleUnits=rad  RotationStandardAxis=+Z  RotationAngle=1.5707963267948968  RotationArbitraryAxis=[0 1 0]  FollAlignAxisA=+X  BaseAlignAxisA=+Y  FollAlignAxisB=+Y  BaseAlignAxisB=+Z  RotationSequenceAxes=FollowerAxes  RotationSequence=XYX  RotationSequenceAngles=[0 0 0]  RotationSequenceAnglesUnits=deg  RotationMatrix=[1 0 0; 0 1 0; 0 0 1]
  Transform9 : sm_lib/Frames and Transforms/Rigid Transform  TranslationMethod=Cartesian  TranslationLengthUnit=mm  TranslationStandardAxis=+Z  TranslationStandardOffset=0  TranslationCartesianOffset=[-25.5 -379.13900000000001 73.075699999999998]  TranslationROffset=0  TranslationROffsetUnits=m  TranslationZOffset=0  TranslationZOffsetUnits=m  TranslationThetaOffset=0  TranslationThetaOffsetUnits=deg  RotationMethod=ArbitraryAxis  RotationAngleUnits=rad  RotationStandardAxis=+Z  RotationAngle=1.5707963267948968  RotationArbitraryAxis=[0 1 0]  FollAlignAxisA=+X  BaseAlignAxisA=+Y  FollAlignAxisB=+Y  BaseAlignAxisB=+Z  RotationSequenceAxes=FollowerAxes  RotationSequence=XYX  RotationSequenceAngles=[0 0 0]  RotationSequenceAnglesUnits=deg  RotationMatrix=[1 0 0; 0 1 0; 0 0 1]
  F : PMIOPort  Port=1  Side=Left
  connections:
  Transform/LConn1 -- ReferenceFrame/RConn1 -- Transform8/LConn1 -- Transform9/LConn1 -- Transform7/LConn1 -- Transform6/LConn1 -- Transform5/LConn1 -- Transform4/LConn1 -- Transform3/LConn1 -- Transform2/LConn1 -- Transform13/LConn1 -- Transform12/LConn1 -- Transform11/LConn1 -- Transform10/LConn1 -- Transform1/LConn1
  Transform/RConn1 -- F/RConn1
  Cavalier_4_RIGID/LConn1 -- Transform9/RConn1
  Faux_flasque_moteur_1_RIGID/LConn1 -- Transform10/RConn1
  Faux_flasque_moteur_2_RIGID/LConn1 -- Transform11/RConn1
  Faux_rotor_1_RIGID/LConn1 -- Transform12/RConn1
  Montant_droit_1_RIGID/LConn1 -- Transform1/RConn1
  Montant_gauche_1_RIGID/LConn1 -- Transform2/RConn1
  Plateau_1_RIGID/LConn1 -- Transform3/RConn1
  Tirant_80_1_RIGID/LConn1 -- Transform4/RConn1
  Tirant_80_2_RIGID/LConn1 -- Transform5/RConn1
  Cavalier_1_RIGID/LConn1 -- Transform6/RConn1
  Cavalier_2_RIGID/LConn1 -- Transform7/RConn1
  Cavalier_3_RIGID/LConn1 -- Transform8/RConn1
  Transform13/RConn1 -- Camera_1_RIGID/LConn1
